simulink model "ExitSendAndTick_2018a"  (R2018a)
settings: Solver=VariableStepAuto  StartTime=0.0  StopTime=10.0  RelTol=1e-3
settings Model: Creator=apple  LastModifiedBy=apple
settings DataIOCC: ReturnWorkspaceOutputs=on
settings SFSimCC: SimUseLocalCustomCode=on
settings RTWCC: RTWUseLocalCustomCode=on

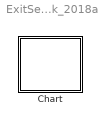
== system ExitSendAndTick_2018a ==
  Chart : Stateflow chart  TreatAsAtomicUnit=on

== stateflow chart ExitSendAndTick_2018a/Chart ==
  state A
    en:fprintf("Entry A");
    du:fprintf("During A");
    ex:fprintf("Exit A");send(F);
    state A1
      en:fprintf("Entry A1");
      du:fprintf("During A1");
      ex:fprintf("Exit A1");
    state A2
      en:fprintf("Entry A2");
      du:fprintf("During A2");
      ex:fprintf("Exit A2");
    (default) -> A1
    A1 -> A2 : F
  state B
    en:fprintf("Entry B");
  (default) -> A
  A -> B : before(3,tick)
  events: F local FUNCTION_CALL_EVENT
